simulink model "exam1_2"  (R2020b)
settings: Solver=VariableStepAuto  StartTime=0.0  StopTime=10.0  RelTol=1e-3
settings Model: Creator=User  LastModifiedBy=User

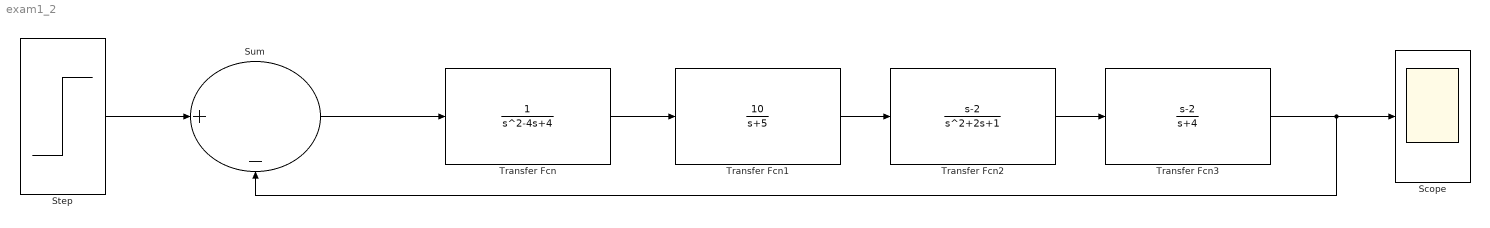
== system exam1_2 ==
  Scope : Scope
  Step : Step  SampleTime=0
  Sum : Sum  Inputs=|+-
  Transfer Fcn : TransferFcn  Denominator=[1 -4 4]
  Transfer Fcn1 : TransferFcn  Numerator=[10]  Denominator=[1 5]
  Transfer Fcn2 : TransferFcn  Numerator=[1 -2]
  Transfer Fcn3 : TransferFcn  Numerator=[1 -2]  Denominator=[1 4]
  wires:
  Sum/1 -> Transfer Fcn/1
  Transfer Fcn/1 -> Transfer Fcn1/1
  Transfer Fcn1/1 -> Transfer Fcn2/1
  Transfer Fcn2/1 -> Transfer Fcn3/1
  Transfer Fcn3/1 -> Sum/2, Scope/1
  Step/1 -> Sum/1
